simulink model "holidays10"  (R2019a)
settings: Solver=VariableStepAuto  StartTime=0.0  StopTime=10.0  RelTol=1e-3
settings Model: Creator=Aditya  LastModifiedBy=Aditya

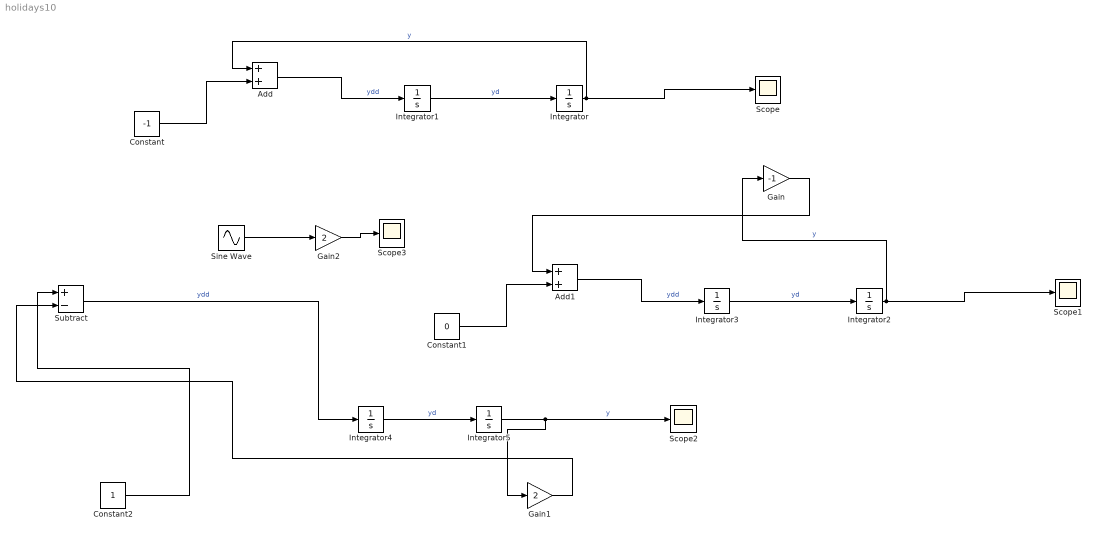
== system holidays10 ==
  Add : Sum
  Add1 : Sum
  Constant : Constant  Value=-1
  Constant1 : Constant  Value=0
  Constant2 : Constant
  Gain : Gain  Gain=-1
  Gain1 : Gain  Gain=2
  Gain2 : Gain  Gain=2
  Integrator{,1..5} (6 alike) : Integrator
  Scope{,1..3} (4 alike) : Scope
  Sine Wave : Sin  SampleTime=0
  Subtract : Sum  Inputs=+-
  wires:
  Add/1 -> Integrator1/1  "ydd"
  Integrator1/1 -> Integrator/1  "yd"
  Integrator/1 -> Add/1, Scope/1  "y"
  Constant/1 -> Add/2
  Add1/1 -> Integrator3/1  "ydd"
  Integrator2/1 -> Gain/1, Scope1/1  "y"
  Integrator3/1 -> Integrator2/1  "yd"
  Constant1/1 -> Add1/2
  Gain/1 -> Add1/1
  Constant2/1 -> Subtract/1
  Subtract/1 -> Integrator4/1  "ydd"
  Integrator4/1 -> Integrator5/1  "yd"
  Integrator5/1 -> Gain1/1, Scope2/1  "y"
  Gain1/1 -> Subtract/2
  Sine Wave/1 -> Gain2/1
  Gain2/1 -> Scope3/1
